simulink model "lo_nhiet"  (R2019a)
settings: Solver=FixedStepAuto  StartTime=0.0  StopTime=1000  FixedStep=1  RelTol=1e-3
libraries: fuzblock x1
settings Model: Creator=ASUS  LastModifiedBy=ASUS

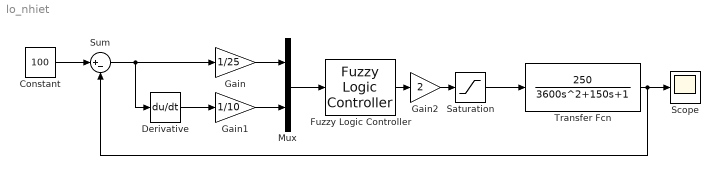
== system lo_nhiet ==
  Constant : Constant  Value=100
  Derivative : Derivative
  Fuzzy Logic Controller : fuzblock/Fuzzy Logic  Controller  FIS='baitap'  OutputSampleNumber=101  DataType=double  FuzzifiedInputs=off  RuleFiringStrengths=off  RuleOutputs=off  AggregatedOutputs=off  SimulateUsing=Interpreted execution  OutOfRangeInputValueMessage=warning  NoRuleFiredMessage=warning  EmptyOutputFuzzySetMessage=warning
  Gain : Gain  Gain=1/25
  Gain1 : Gain  Gain=1/10
  Gain2 : Gain  Gain=2
  Mux : Mux  Inputs=2
  Saturation : Saturate  UpperLimit=1
  Scope : Scope
  Sum : Sum  Inputs=|+-
  Transfer Fcn : TransferFcn  Numerator=[250]  Denominator=[3600 150 1]
  wires:
  Sum/1 -> Derivative/1, Gain/1
  Constant/1 -> Sum/1
  Derivative/1 -> Gain1/1
  Gain/1 -> Mux/1
  Gain1/1 -> Mux/2
  Mux/1 -> Fuzzy Logic Controller/1
  Fuzzy Logic Controller/1 -> Gain2/1
  Transfer Fcn/1 -> Sum/2, Scope/1
  Gain2/1 -> Saturation/1
  Saturation/1 -> Transfer Fcn/1
